simulink model "PTControl"  (Simulink 10.3)
settings: Solver=ode45  StartTime=0.0  StopTime=inf  RelTol=1e-3  EnableMultiTasking=on
(part 2 of 5)

== system PTControl/CarMaker/IPG Vehicle/CarAndTrailer/Forces/Tires ==
  note: The TireXX_Out signals will only be used if FileIdent is "CarMaker-Tire-CM4SL" in the tire parameter file!
      | An example parameter file can be found in Data/Tire/DT_CM4SL_UserTire.
  Sync_In : Inport
  TireFL_In : Inport  Port=2
  TireFR_In : Inport  Port=3
  TireRL_In : Inport  Port=4
  TireRR_In : Inport  Port=5
  Bus Creator{1..4} (4 alike) : BusCreator  Inputs=11
  Demux{1..3,8} (4 alike) : Demux  Outputs=7
      settings: DisplayOption=none
  TireFL : Subsystem
  TireFR : Subsystem
  TireRL : Subsystem
  TireRR : Subsystem
  TireFL_Out : Outport  VectorParamsAs1DForOutWhenUnconnected=off
  TireFR_Out : Outport  Port=2  VectorParamsAs1DForOutWhenUnconnected=off
  TireRL_Out : Outport  Port=3  VectorParamsAs1DForOutWhenUnconnected=off
  TireRR_Out : Outport  Port=4  VectorParamsAs1DForOutWhenUnconnected=off
  wires:
  Sync_In/1 -> TireRR/1(Sync_In), TireRL/1(Sync_In), TireFR/1(Sync_In), TireFL/1(Sync_In)
  Bus Creator4/1 -> TireRR_Out/1
  Bus Creator2/1 -> TireRL_Out/1
  Bus Creator1/1 -> TireFR_Out/1
  Demux3/5 -> TireRR/6(Rim_turnv)  "Tire_In Rim_turnv"
  Demux3/4 -> TireRR/5(Rim_rotv)  "Tire_In Rim_rotv"
  Demux3/1 -> TireRR/2(Load)  "Tire_In Load"
  Demux3/7 -> TireRR/8(muRoad)  "Tire_In mu"
  Demux3/6 -> TireRR/7(InclinAngle)  "Tire_In Camber"
  Demux3/2 -> TireRR/3(vxtrans)  "Tire_In vxtrans"
  Demux3/3 -> TireRR/4(vytrans)  "Tire_In vytrans"
  TireRR/11(AlignTrq) -> Bus Creator4/11  "Tire_Out AlignTrq"
  TireRR/10(RollResist) -> Bus Creator4/10  "Tire_Out RollResist"
  TireRR/9(OverturnTrq) -> Bus Creator4/9  "Tire_Out OverturnTrq"
  TireRR/8(LoadFrc) -> Bus Creator4/8  "Tire_Out LoadFrc"
  TireRR/7(SideFrc) -> Bus Creator4/7  "Tire_Out SideFrc"
  TireRR/6(LongFrc) -> Bus Creator4/6  "Tire_Out LongFrc"
  TireRR/5(vBelt) -> Bus Creator4/5  "Tire_Out vBelt"
  TireRR/4(rBelt_eff) -> Bus Creator4/4  "Tire_Out rBelt_eff"
  TireRR/3(TurnSlp) -> Bus Creator4/3  "Tire_Out TurnSlp"
  TireRR/1(Slp) -> Bus Creator4/1  "Tire_Out Slp"
  TireRR/2(Alpha) -> Bus Creator4/2  "Tire_Out Alpha"
  Demux2/5 -> TireRL/6(Rim_turnv)  "Tire_In Rim_turnv"
  Demux2/4 -> TireRL/5(Rim_rotv)  "Tire_In Rim_rotv"
  Demux2/1 -> TireRL/2(Load)  "Tire_In Load"
  Demux2/7 -> TireRL/8(muRoad)  "Tire_In mu"
  Demux2/6 -> TireRL/7(InclinAngle)  "Tire_In Camber"
  Demux2/2 -> TireRL/3(vxtrans)  "Tire_In vxtrans"
  Demux2/3 -> TireRL/4(vytrans)  "Tire_In vytrans"
  TireRL/11(AlignTrq) -> Bus Creator2/11  "Tire_Out AlignTrq"
  TireRL/10(RollResist) -> Bus Creator2/10  "Tire_Out RollResist"
  TireRL/9(OverturnTrq) -> Bus Creator2/9  "Tire_Out OverturnTrq"
  TireRL/8(LoadFrc) -> Bus Creator2/8  "Tire_Out LoadFrc"
  TireRL/7(SideFrc) -> Bus Creator2/7  "Tire_Out SideFrc"
  TireRL/6(LongFrc) -> Bus Creator2/6  "Tire_Out LongFrc"
  TireRL/5(vBelt) -> Bus Creator2/5  "Tire_Out vBelt"
  TireRL/4(rBelt_eff) -> Bus Creator2/4  "Tire_Out rBelt_eff"
  TireRL/3(TurnSlp) -> Bus Creator2/3  "Tire_Out TurnSlp"
  TireRL/1(Slp) -> Bus Creator2/1  "Tire_Out Slp"
  TireRL/2(Alpha) -> Bus Creator2/2  "Tire_Out Alpha"
  Demux1/5 -> TireFR/6(Rim_turnv)  "Tire_In Rim_turnv"
  Demux1/4 -> TireFR/5(Rim_rotv)  "Tire_In Rim_rotv"
  Demux1/1 -> TireFR/2(Load)  "Tire_In Load"
  Demux1/7 -> TireFR/8(muRoad)  "Tire_In mu"
  Demux1/6 -> TireFR/7(InclinAngle)  "Tire_In Camber"
  Demux1/2 -> TireFR/3(vxtrans)  "Tire_In vxtrans"
  Demux1/3 -> TireFR/4(vytrans)  "Tire_In vytrans"
  TireFR/11(AlignTrq) -> Bus Creator1/11  "Tire_Out AlignTrq"
  TireFR/10(RollResist) -> Bus Creator1/10  "Tire_Out RollResist"
  TireFR/9(OverturnTrq) -> Bus Creator1/9  "Tire_Out OverturnTrq"
  TireFR/8(LoadFrc) -> Bus Creator1/8  "Tire_Out LoadFrc"
  TireFR/7(SideFrc) -> Bus Creator1/7  "Tire_Out SideFrc"
  TireFR/6(LongFrc) -> Bus Creator1/6  "Tire_Out LongFrc"
  TireFR/5(vBelt) -> Bus Creator1/5  "Tire_Out vBelt"
  TireFR/4(rBelt_eff) -> Bus Creator1/4  "Tire_Out rBelt_eff"
  TireFR/3(TurnSlp) -> Bus Creator1/3  "Tire_Out TurnSlp"
  TireFR/1(Slp) -> Bus Creator1/1  "Tire_Out Slp"
  TireFR/2(Alpha) -> Bus Creator1/2  "Tire_Out Alpha"
  Demux8/5 -> TireFL/6(Rim_turnv)  "Tire_In Rim_turnv"
  Demux8/4 -> TireFL/5(Rim_rotv)  "Tire_In Rim_rotv"
  TireFL_In/1 -> Demux8/1
  Demux8/1 -> TireFL/2(Load)  "Tire_In Load"
  Demux8/7 -> TireFL/8(muRoad)  "Tire_In mu"
  Demux8/6 -> TireFL/7(InclinAngle)  "Tire_In Camber"
  Demux8/2 -> TireFL/3(vxtrans)  "Tire_In vxtrans"
  Demux8/3 -> TireFL/4(vytrans)  "Tire_In vytrans"
  TireFL/11(AlignTrq) -> Bus Creator3/11  "Tire_Out AlignTrq"
  TireFL/10(RollResist) -> Bus Creator3/10  "Tire_Out RollResist"
  TireFL/9(OverturnTrq) -> Bus Creator3/9  "Tire_Out OverturnTrq"
  TireFL/8(LoadFrc) -> Bus Creator3/8  "Tire_Out LoadFrc"
  TireFL/7(SideFrc) -> Bus Creator3/7  "Tire_Out SideFrc"
  TireFL/6(LongFrc) -> Bus Creator3/6  "Tire_Out LongFrc"
  TireFL/5(vBelt) -> Bus Creator3/5  "Tire_Out vBelt"
  TireFL/4(rBelt_eff) -> Bus Creator3/4  "Tire_Out rBelt_eff"
  TireFL/3(TurnSlp) -> Bus Creator3/3  "Tire_Out TurnSlp"
  TireFL/1(Slp) -> Bus Creator3/1  "Tire_Out Slp"
  TireFL/2(Alpha) -> Bus Creator3/2  "Tire_Out Alpha"
  Bus Creator3/1 -> TireFL_Out/1
  TireFR_In/1 -> Demux1/1
  TireRL_In/1 -> Demux2/1
  TireRR_In/1 -> Demux3/1

== system PTControl/CarMaker/IPG Vehicle/CarAndTrailer/Forces/Vehicle Forces ==
  Sync_In : Inport
  Bus Creator1 : BusCreator  Inputs=12
  Bus Creator8 : BusCreator  Inputs=16
  BusCreator1 : BusCreator  Inputs=4
  BusCreator2 : BusCreator  Inputs=9
  Demux : Demux  Outputs=16
      settings: DisplayOption=none
  Demux1 : Demux  Outputs=12
      settings: DisplayOption=none
  Demux2 : Demux  Outputs=13
      settings: DisplayOption=none
  Forces : S-Function  FunctionName=CM_Sfun  Parameters='Forces'  SFunctionDeploymentMode=off  EnableBusSupport=off
  Terminator : Terminator
  Sync_Out : Outport  VectorParamsAs1DForOutWhenUnconnected=off
  Car.Virtual : Outport  Port=2  VectorParamsAs1DForOutWhenUnconnected=off
  Car.Aero : Outport  Port=3  VectorParamsAs1DForOutWhenUnconnected=off
  Car.Load : Outport  Port=4  VectorParamsAs1DForOutWhenUnconnected=off
  wires:
  BusCreator1/1 -> Terminator/1  "Aero IF (in)"
  Demux2/13 -> BusCreator2/9  "car Aero Trq_1 z"
  Demux2/12 -> BusCreator2/8  "car Aero Trq_1 y"
  Demux2/11 -> BusCreator2/7  "car Aero Trq_1 x"
  Demux2/10 -> BusCreator2/6  "car Aero Frc_1 z"
  Demux2/9 -> BusCreator2/5  "car Aero Frc_1 y"
  Demux2/8 -> BusCreator2/4  "car Aero Frc_1 x"
  Demux2/7 -> BusCreator2/3  "car Aero PoA_1 z"
  Demux2/6 -> BusCreator2/2  "car Aero PoA_1 y"
  Demux2/5 -> BusCreator2/1  "car Aero PoA_1 x"
  Demux2/4 -> BusCreator1/4  "car Aero tau_1"
  Demux2/3 -> BusCreator1/3  "car Aero ApproachVel_1 z"
  Demux2/2 -> BusCreator1/2  "car Aero ApproachVel_1 y"
  Demux2/1 -> BusCreator1/1  "car Aero ApproachVel_1 x"
  Demux/16 -> Bus Creator8/16  "Car Load_3 tz"
  Demux/15 -> Bus Creator8/15  "Car Load_3 ty"
  Demux/14 -> Bus Creator8/14  "Car Load_3 tx"
  Demux/13 -> Bus Creator8/13  "Car Load_3 mass"
  Demux1/12 -> Bus Creator1/12  "Car Virtual Trq_0 z"
  Demux1/11 -> Bus Creator1/11  "Car Virtual Trq_0 y"
  Demux1/10 -> Bus Creator1/10  "Car Virtual Trq_0 x"
  Demux1/9 -> Bus Creator1/9  "Car Virtual Trq_1 z"
  Demux1/8 -> Bus Creator1/8  "Car Virtual Trq_1 y"
  Demux1/7 -> Bus Creator1/7  "Car Virtual Trq_1 x"
  Demux1/6 -> Bus Creator1/6  "Car Virtual Frc_0 z"
  Demux1/5 -> Bus Creator1/5  "Car Virtual Frc_0 y"
  Demux1/4 -> Bus Creator1/4  "Car Virtual Frc_0 x"
  Sync_In/1 -> Forces/1
  Forces/1 -> Sync_Out/1
  BusCreator2/1 -> Car.Aero/1
  Demux1/1 -> Bus Creator1/1  "Car Virtual Frc_1 x"
  Demux1/2 -> Bus Creator1/2  "Car Virtual Frc_1 y"
  Demux1/3 -> Bus Creator1/3  "Car Virtual Frc_1 z"
  Forces/3 -> Demux2/1
  Forces/2 -> Demux1/1
  Bus Creator1/1 -> Car.Virtual/1
  Bus Creator8/1 -> Car.Load/1
  Demux/1 -> Bus Creator8/1  "Car Load_0 mass"
  Demux/2 -> Bus Creator8/2  "Car Load_0 tx"
  Demux/3 -> Bus Creator8/3  "Car Load_0 ty"
  Demux/4 -> Bus Creator8/4  "Car Load_0 tz"
  Demux/5 -> Bus Creator8/5  "Car Load_1 mass"
  Demux/6 -> Bus Creator8/6  "Car Load_1 tx"
  Demux/7 -> Bus Creator8/7  "Car Load_1 ty"
  Demux/8 -> Bus Creator8/8  "Car Load_1 tz"
  Demux/9 -> Bus Creator8/9  "Car Load_2 mass"
  Demux/10 -> Bus Creator8/10  "Car Load_2 tx"
  Demux/11 -> Bus Creator8/11  "Car Load_2 ty"
  Demux/12 -> Bus Creator8/12  "Car Load_2 tz"
  Forces/4 -> Demux/1

== system PTControl/CarMaker/IPG Vehicle/CarAndTrailer/Trailer/CreateBus Car.Hitch.FrcTrq ==
  In1 : Inport
  Bus Creator7 : BusCreator  Inputs=6
  Demux7 : Demux  Outputs=6
      settings: DisplayOption=none
  Out1 : Outport  VectorParamsAs1DForOutWhenUnconnected=off
  wires:
  In1/1 -> Demux7/1
  Bus Creator7/1 -> Out1/1
  Demux7/6 -> Bus Creator7/6  "Car Hitch Trq2Car z"
  Demux7/5 -> Bus Creator7/5  "Car Hitch Trq2Car y"
  Demux7/4 -> Bus Creator7/4  "Car Hitch Trq2Car x"
  Demux7/3 -> Bus Creator7/3  "Car Hitch Frc2Car z"
  Demux7/2 -> Bus Creator7/2  "Car Hitch Frc2Car y"
  Demux7/1 -> Bus Creator7/1  "Car Hitch Frc2Car x"

== system PTControl/CarMaker/IPG Vehicle/CarAndTrailer/Trailer/CreateBus Vhcl.Motion ==
  In1 : Inport
  BusCreator : BusCreator  Inputs=15
  Demux : Demux  Outputs=15
      settings: DisplayOption=none
  Out1 : Outport  VectorParamsAs1DForOutWhenUnconnected=off
  wires:
  Demux/15 -> BusCreator/15  "Vhcl YawAcc"
  Demux/14 -> BusCreator/14  "Vhcl YawVel"
  Demux/13 -> BusCreator/13  "Vhcl Yaw"
  Demux/12 -> BusCreator/12  "Vhcl PitchAcc"
  Demux/11 -> BusCreator/11  "Vhcl PitchVel"
  Demux/10 -> BusCreator/10  "Vhcl Pitch"
  Demux/9 -> BusCreator/9  "Vhcl RollAcc"
  Demux/8 -> BusCreator/8  "Vhcl RollVel"
  Demux/7 -> BusCreator/7  "Vhcl Roll"
  Demux/6 -> BusCreator/6  "Vhcl Hitch_Pos z"
  Demux/5 -> BusCreator/5  "Vhcl Hitch_Pos y"
  Demux/4 -> BusCreator/4  "Vhcl Hitch_Pos x"
  Demux/3 -> BusCreator/3  "Vhcl sRoad"
  Demux/2 -> BusCreator/2  "Vhcl Distance"
  Demux/1 -> BusCreator/1  "Vhcl v"
  In1/1 -> Demux/1
  BusCreator/1 -> Out1/1

== system PTControl/CarMaker/IPG Vehicle/CarAndTrailer/Trailer/CreateBus Vhcl.PoI ==
  In1 : Inport
  Bus Creator3 : BusCreator  Inputs=18
  Demux3 : Demux  Outputs=18
      settings: DisplayOption=none
  Out1 : Outport  VectorParamsAs1DForOutWhenUnconnected=off
  wires:
  Demux3/18 -> Bus Creator3/18  "Vhcl PoI_GCS Elev"
  Demux3/17 -> Bus Creator3/17  "Vhcl PoI_GCS Lat"
  Demux3/16 -> Bus Creator3/16  "Vhcl PoI_GCS Long"
  Demux3/15 -> Bus Creator3/15  "Vhcl PoI_Acc_1 z"
  Demux3/14 -> Bus Creator3/14  "Vhcl PoI_Acc_1 y"
  Demux3/13 -> Bus Creator3/13  "Vhcl PoI_Acc_1 x"
  Demux3/12 -> Bus Creator3/12  "Vhcl PoI_Vel_1 z"
  Demux3/11 -> Bus Creator3/11  "Vhcl PoI_Vel_1 y"
  Demux3/10 -> Bus Creator3/10  "Vhcl PoI_Vel_1 x"
  Demux3/9 -> Bus Creator3/9  "Vhcl PoI_Acc z"
  Demux3/8 -> Bus Creator3/8  "Vhcl PoI_Acc y"
  Demux3/7 -> Bus Creator3/7  "Vhcl PoI_Acc x"
  Demux3/6 -> Bus Creator3/6  "Vhcl PoI_Vel z"
  Demux3/5 -> Bus Creator3/5  "Vhcl PoI_Vel y"
  Demux3/4 -> Bus Creator3/4  "Vhcl PoI_Vel x"
  Demux3/3 -> Bus Creator3/3  "Vhcl PoI_Pos z"
  Demux3/2 -> Bus Creator3/2  "Vhcl PoI_Pos y"
  In1/1 -> Demux3/1
  Bus Creator3/1 -> Out1/1
  Demux3/1 -> Bus Creator3/1  "Vhcl PoI_Pos x"

== system PTControl/CarMaker/IPG Vehicle/CarAndTrailer/Trailer/CreateBus Vhcl.Steering ==
  In1 : Inport
  Bus Creator3 : BusCreator  Inputs=4
  Demux : Demux
      settings: DisplayOption=none
  Out1 : Outport  VectorParamsAs1DForOutWhenUnconnected=off
  wires:
  Bus Creator3/1 -> Out1/1
  Demux/1 -> Bus Creator3/1  "Vhcl Steering Ang"
  Demux/3 -> Bus Creator3/3  "Vhcl Steering AngAcc"
  Demux/2 -> Bus Creator3/2  "Vhcl Steering AngVel"
  Demux/4 -> Bus Creator3/4  "Vhcl Steering Trq"
  In1/1 -> Demux/1

== system PTControl/CarMaker/IPG Vehicle/CarAndTrailer/Trailer/CreateBus Vhcl.Wheel.FL ==
  In1 : Inport
  Bus Creator3 : BusCreator  Inputs=14
  Demux3 : Demux  Outputs=14
      settings: DisplayOption=none
  Out1 : Outport  VectorParamsAs1DForOutWhenUnconnected=off
  wires:
  Demux3/14 -> Bus Creator3/14  "Vhcl Wheel FL Trq_WhlBearing"
  Demux3/13 -> Bus Creator3/13  "Vhcl Wheel FL Trq_T2W"
  Demux3/12 -> Bus Creator3/12  "Vhcl Wheel FL SideSlip"
  Demux3/11 -> Bus Creator3/11  "Vhcl Wheel FL LongSlip"
  Demux3/10 -> Bus Creator3/10  "Vhcl Wheel FL vBelt"
  Demux3/9 -> Bus Creator3/9  "Vhcl Wheel FL Fz"
  Demux3/8 -> Bus Creator3/8  "Vhcl Wheel FL Fy"
  Demux3/7 -> Bus Creator3/7  "Vhcl Wheel FL Fx"
  Demux3/6 -> Bus Creator3/6  "Vhcl Wheel FL r_zxy z"
  Demux3/5 -> Bus Creator3/5  "Vhcl Wheel FL r_zxy y"
  Demux3/4 -> Bus Creator3/4  "Vhcl Wheel FL r_zxy x"
  Demux3/3 -> Bus Creator3/3  "Vhcl Wheel FL t z"
  Demux3/2 -> Bus Creator3/2  "Vhcl Wheel FL t y"
  In1/1 -> Demux3/1
  Bus Creator3/1 -> Out1/1
  Demux3/1 -> Bus Creator3/1  "Vhcl Wheel FL t x"

== system PTControl/CarMaker/IPG Vehicle/CarAndTrailer/Trailer/CreateBus Vhcl.Wheel.FR ==
  In1 : Inport
  Bus Creator3 : BusCreator  Inputs=14
  Demux3 : Demux  Outputs=14
      settings: DisplayOption=none
  Out1 : Outport  VectorParamsAs1DForOutWhenUnconnected=off
  wires:
  Demux3/14 -> Bus Creator3/14  "Vhcl Wheel FR Trq_WhlBearing"
  Demux3/13 -> Bus Creator3/13  "Vhcl Wheel FR Trq_T2W"
  Demux3/12 -> Bus Creator3/12  "Vhcl Wheel FR SideSlip"
  Demux3/11 -> Bus Creator3/11  "Vhcl Wheel FR LongSlip"
  Demux3/10 -> Bus Creator3/10  "Vhcl Wheel FR vBelt"
  Demux3/9 -> Bus Creator3/9  "Vhcl Wheel FR Fz"
  Demux3/8 -> Bus Creator3/8  "Vhcl Wheel FR Fy"
  Demux3/7 -> Bus Creator3/7  "Vhcl Wheel FR Fx"
  Demux3/6 -> Bus Creator3/6  "Vhcl Wheel FR r_zxy z"
  Demux3/5 -> Bus Creator3/5  "Vhcl Wheel FR r_zxy y"
  Demux3/4 -> Bus Creator3/4  "Vhcl Wheel FR r_zxy x"
  Demux3/3 -> Bus Creator3/3  "Vhcl Wheel FR t z"
  Demux3/2 -> Bus Creator3/2  "Vhcl Wheel FR t y"
  In1/1 -> Demux3/1
  Bus Creator3/1 -> Out1/1
  Demux3/1 -> Bus Creator3/1  "Vhcl Wheel FR t x"

== system PTControl/CarMaker/IPG Vehicle/CarAndTrailer/Trailer/CreateBus Vhcl.Wheel.RL ==
  In1 : Inport
  Bus Creator3 : BusCreator  Inputs=14
  Demux3 : Demux  Outputs=14
      settings: DisplayOption=none
  Out1 : Outport  VectorParamsAs1DForOutWhenUnconnected=off
  wires:
  Demux3/14 -> Bus Creator3/14  "Vhcl Wheel RL Trq_WhlBearing"
  Demux3/13 -> Bus Creator3/13  "Vhcl Wheel RL Trq_T2W"
  Demux3/12 -> Bus Creator3/12  "Vhcl Wheel RL SideSlip"
  Demux3/11 -> Bus Creator3/11  "Vhcl Wheel RL LongSlip"
  Demux3/10 -> Bus Creator3/10  "Vhcl Wheel RL vBelt"
  Demux3/9 -> Bus Creator3/9  "Vhcl Wheel RL Fz"
  Demux3/8 -> Bus Creator3/8  "Vhcl Wheel RL Fy"
  Demux3/7 -> Bus Creator3/7  "Vhcl Wheel RL Fx"
  Demux3/6 -> Bus Creator3/6  "Vhcl Wheel RL r_zxy z"
  Demux3/5 -> Bus Creator3/5  "Vhcl Wheel RL r_zxy y"
  Demux3/4 -> Bus Creator3/4  "Vhcl Wheel RL r_zxy x"
  Demux3/3 -> Bus Creator3/3  "Vhcl Wheel RL t z"
  Demux3/2 -> Bus Creator3/2  "Vhcl Wheel RL t y"
  In1/1 -> Demux3/1
  Bus Creator3/1 -> Out1/1
  Demux3/1 -> Bus Creator3/1  "Vhcl Wheel RL t x"

== system PTControl/CarMaker/IPG Vehicle/CarAndTrailer/Trailer/CreateBus Vhcl.Wheel.RR ==
  In1 : Inport
  Bus Creator3 : BusCreator  Inputs=14
  Demux3 : Demux  Outputs=14
      settings: DisplayOption=none
  Out1 : Outport  VectorParamsAs1DForOutWhenUnconnected=off
  wires:
  Demux3/14 -> Bus Creator3/14  "Vhcl Wheel RR Trq_WhlBearing"
  Demux3/13 -> Bus Creator3/13  "Vhcl Wheel RR Trq_T2W"
  Demux3/12 -> Bus Creator3/12  "Vhcl Wheel RR SideSlip"
  Demux3/11 -> Bus Creator3/11  "Vhcl Wheel RR LongSlip"
  Demux3/10 -> Bus Creator3/10  "Vhcl Wheel RR vBelt"
  Demux3/9 -> Bus Creator3/9  "Vhcl Wheel RR Fz"
  Demux3/8 -> Bus Creator3/8  "Vhcl Wheel RR Fy"
  Demux3/7 -> Bus Creator3/7  "Vhcl Wheel RR Fx"
  Demux3/6 -> Bus Creator3/6  "Vhcl Wheel RR r_zxy z"
  Demux3/5 -> Bus Creator3/5  "Vhcl Wheel RR r_zxy y"
  Demux3/4 -> Bus Creator3/4  "Vhcl Wheel RR r_zxy x"
  Demux3/3 -> Bus Creator3/3  "Vhcl Wheel RR t z"
  Demux3/2 -> Bus Creator3/2  "Vhcl Wheel RR t y"
  In1/1 -> Demux3/1
  Bus Creator3/1 -> Out1/1
  Demux3/1 -> Bus Creator3/1  "Vhcl Wheel RR t x"

== system PTControl/CarMaker/IPG Vehicle/PowerTrain/PTControl Example/CreateBus PTC BatteryHVOut ==
  In : Inport
  BusCreator : BusCreator  Inputs=2
  Demux : Demux  Outputs=2
      settings: DisplayOption=none
  Out : Outport  VectorParamsAs1DForOutWhenUnconnected=off
  wires:
  Demux/2 -> BusCreator/2  "PTC BattHVOut MassFlowCool_trg"
  Demux/1 -> BusCreator/1  "PTC BattHVOut Temp_trg"
  In/1 -> Demux/1
  BusCreator/1 -> Out/1

== system PTControl/CarMaker/IPG Vehicle/PowerTrain/PTControl Example/CreateBus PTC BatteryLVOut ==
  In : Inport
  BusCreator : BusCreator  Inputs=2
  Demux : Demux  Outputs=2
      settings: DisplayOption=none
  Out : Outport  VectorParamsAs1DForOutWhenUnconnected=off
  wires:
  Demux/2 -> BusCreator/2  "PTC BattLVOut MassFlowCool_trg"
  In/1 -> Demux/1
  Demux/1 -> BusCreator/1  "PTC BattLVOut Temp_trg"
  BusCreator/1 -> Out/1

== system PTControl/CarMaker/IPG Vehicle/PowerTrain/PTControl Example/CreateBus PTC EngineOut ==
  In : Inport
  BusCreator : BusCreator  Inputs=5
  Demux : Demux  Outputs=5
      settings: DisplayOption=none
  Out : Outport  VectorParamsAs1DForOutWhenUnconnected=off
  wires:
  Demux/5 -> BusCreator/5  "PTC EngineOut rotv_trg"
  Demux/4 -> BusCreator/4  "PTC EngineOut Trq_trg"
  Demux/3 -> BusCreator/3  "PTC EngineOut Load"
  Demux/2 -> BusCreator/2  "PTC EngineOut FuelCutOff"
  Demux/1 -> BusCreator/1  "PTC EngineOut set_ISC"
  BusCreator/1 -> Out/1
  In/1 -> Demux/1

== system PTControl/CarMaker/IPG Vehicle/PowerTrain/PTControl Example/CreateBus PTC ISGOut ==
  In : Inport
  BusCreator : BusCreator  Inputs=3
  Demux : Demux  Outputs=3
      settings: DisplayOption=none
  Out : Outport  VectorParamsAs1DForOutWhenUnconnected=off
  wires:
  Demux/3 -> BusCreator/3  "PTC ISGOut rotv_trg"
  Demux/2 -> BusCreator/2  "PTC ISGOut Trq_trg"
  Demux/1 -> BusCreator/1  "PTC ISGOut Load"
  BusCreator/1 -> Out/1
  In/1 -> Demux/1

== system PTControl/CarMaker/IPG Vehicle/PowerTrain/PTControl Example/CreateBus PTC MiscOut ==
  In : Inport
  BusCreator : BusCreator  Inputs=4
  Demux : Demux
      settings: DisplayOption=none
  Out : Outport  VectorParamsAs1DForOutWhenUnconnected=off
  wires:
  Demux/4 -> BusCreator/4  "PTC_Out Ignition"
  Demux/3 -> BusCreator/3  "PTC_Out StrategyMode"
  Demux/2 -> BusCreator/2  "PTC_Out OperationError"
  Demux/1 -> BusCreator/1  "PTC_Out OperationState"
  BusCreator/1 -> Out/1
  In/1 -> Demux/1

== system PTControl/CarMaker/IPG Vehicle/PowerTrain/PTControl Example/CreateBus PTC PwrSupplyOut ==
  In : Inport
  BusCreator : BusCreator  Inputs=1
  Demux : Demux  Outputs=1
      settings: DisplayOption=none
  Out : Outport  VectorParamsAs1DForOutWhenUnconnected=off
  wires:
  Demux/1 -> BusCreator/1  "PTC PwrSupplyOut Pwr_HV1toLV_trg"
  BusCreator/1 -> Out/1
  In/1 -> Demux/1

== system PTControl/CarMaker/IPG Vehicle/PowerTrain/PTControl Example/CreateBus PTC WheelOut ==
  In : Inport
  BusCreator : BusCreator  Inputs=8
  Demux : Demux  Outputs=8
      settings: DisplayOption=none
  Out : Outport  VectorParamsAs1DForOutWhenUnconnected=off
  wires:
  Demux/8 -> BusCreator/8  "PTC WheelOut_RR Trq_BrakeReg_max"
  Demux/7 -> BusCreator/7  "PTC WheelOut_RR Trq_BrakeReg"
  Demux/6 -> BusCreator/6  "PTC WheelOut_RL Trq_BrakeReg_max"
  Demux/5 -> BusCreator/5  "PTC WheelOut_RL Trq_BrakeReg"
  Demux/4 -> BusCreator/4  "PTC WheelOut_FR Trq_BrakeReg_max"
  Demux/3 -> BusCreator/3  "PTC WheelOut_FR Trq_BrakeReg"
  Demux/2 -> BusCreator/2  "PTC WheelOut_FL Trq_BrakeReg_max"
  Demux/1 -> BusCreator/1  "PTC WheelOut_FL Trq_BrakeReg"
  BusCreator/1 -> Out/1
  In/1 -> Demux/1

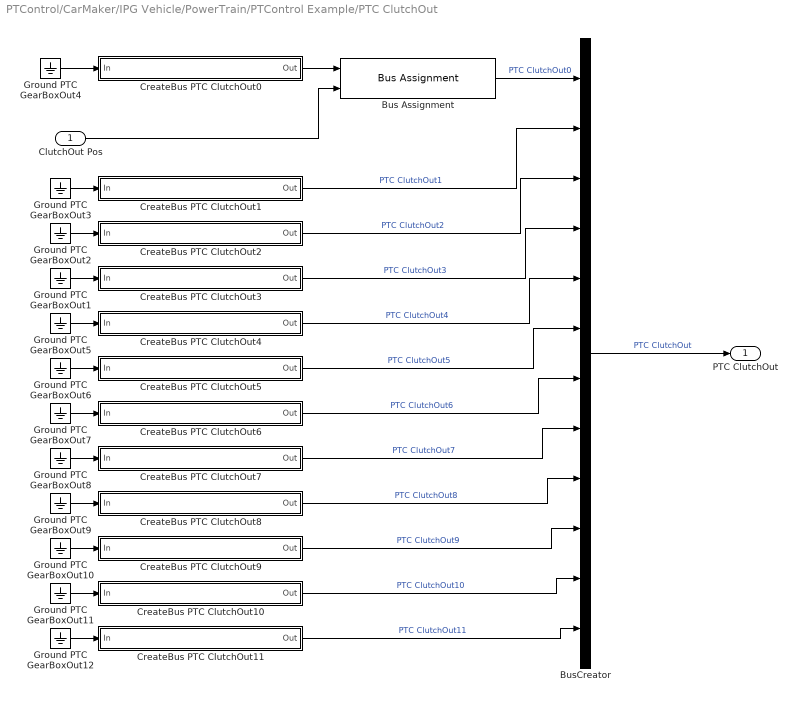
== system PTControl/CarMaker/IPG Vehicle/PowerTrain/PTControl Example/PTC ClutchOut ==
  ClutchOut Pos : Inport
  Bus Assignment : BusAssignment  AssignedSignals=PTC ClutchOut0 Pos
  BusCreator : BusCreator  Inputs=12
  CreateBus PTC ClutchOut0 : Subsystem
  CreateBus PTC ClutchOut1 : Subsystem
  CreateBus PTC ClutchOut10 : Subsystem
  CreateBus PTC ClutchOut11 : Subsystem
  CreateBus PTC ClutchOut2 : Subsystem
  CreateBus PTC ClutchOut3 : Subsystem
  CreateBus PTC ClutchOut4 : Subsystem
  CreateBus PTC ClutchOut5 : Subsystem
  CreateBus PTC ClutchOut6 : Subsystem
  CreateBus PTC ClutchOut7 : Subsystem
  CreateBus PTC ClutchOut8 : Subsystem
  CreateBus PTC ClutchOut9 : Subsystem
  Ground PTC GearBoxOut{1..12} (12 alike) : Ground
  PTC ClutchOut : Outport
  wires:
  ClutchOut Pos/1 -> Bus Assignment/2
  CreateBus PTC ClutchOut0/1(Out) -> Bus Assignment/1
  Ground PTC GearBoxOut4/1 -> CreateBus PTC ClutchOut0/1(In)
  Ground PTC GearBoxOut3/1 -> CreateBus PTC ClutchOut1/1(In)
  Ground PTC GearBoxOut2/1 -> CreateBus PTC ClutchOut2/1(In)
  Ground PTC GearBoxOut1/1 -> CreateBus PTC ClutchOut3/1(In)
  Ground PTC GearBoxOut5/1 -> CreateBus PTC ClutchOut4/1(In)
  Ground PTC GearBoxOut6/1 -> CreateBus PTC ClutchOut5/1(In)
  Ground PTC GearBoxOut7/1 -> CreateBus PTC ClutchOut6/1(In)
  Ground PTC GearBoxOut8/1 -> CreateBus PTC ClutchOut7/1(In)
  Ground PTC GearBoxOut9/1 -> CreateBus PTC ClutchOut8/1(In)
  Ground PTC GearBoxOut10/1 -> CreateBus PTC ClutchOut9/1(In)
  Ground PTC GearBoxOut11/1 -> CreateBus PTC ClutchOut10/1(In)
  Ground PTC GearBoxOut12/1 -> CreateBus PTC ClutchOut11/1(In)
  Bus Assignment/1 -> BusCreator/1  "PTC ClutchOut0"
  CreateBus PTC ClutchOut1/1(Out) -> BusCreator/2  "PTC ClutchOut1"
  CreateBus PTC ClutchOut2/1(Out) -> BusCreator/3  "PTC ClutchOut2"
  CreateBus PTC ClutchOut3/1(Out) -> BusCreator/4  "PTC ClutchOut3"
  CreateBus PTC ClutchOut4/1(Out) -> BusCreator/5  "PTC ClutchOut4"
  CreateBus PTC ClutchOut5/1(Out) -> BusCreator/6  "PTC ClutchOut5"
  CreateBus PTC ClutchOut6/1(Out) -> BusCreator/7  "PTC ClutchOut6"
  CreateBus PTC ClutchOut7/1(Out) -> BusCreator/8  "PTC ClutchOut7"
  CreateBus PTC ClutchOut8/1(Out) -> BusCreator/9  "PTC ClutchOut8"
  CreateBus PTC ClutchOut9/1(Out) -> BusCreator/10  "PTC ClutchOut9"
  CreateBus PTC ClutchOut10/1(Out) -> BusCreator/11  "PTC ClutchOut10"
  CreateBus PTC ClutchOut11/1(Out) -> BusCreator/12  "PTC ClutchOut11"
  BusCreator/1 -> PTC ClutchOut/1  "PTC ClutchOut"

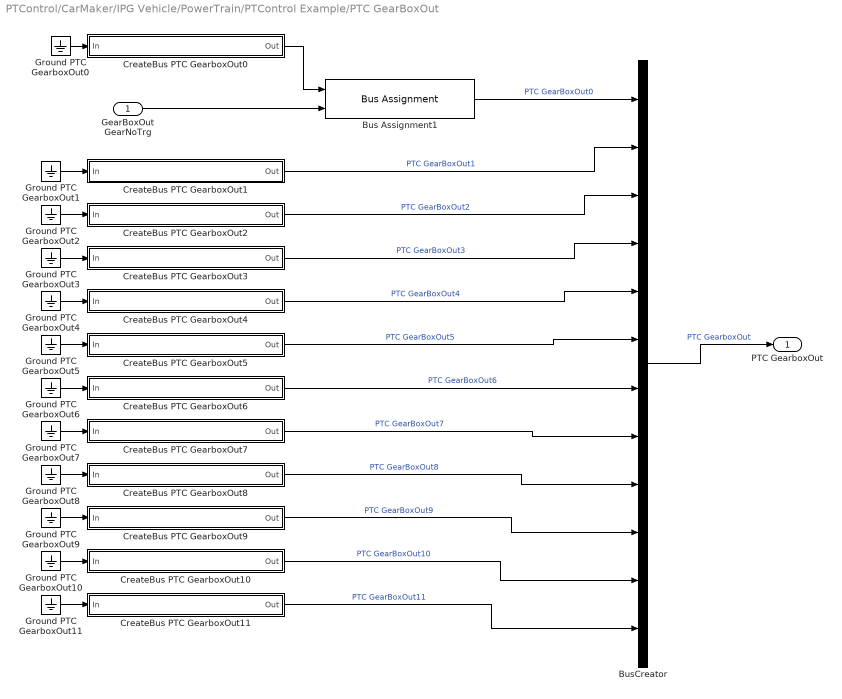
== system PTControl/CarMaker/IPG Vehicle/PowerTrain/PTControl Example/PTC GearBoxOut ==
  GearBoxOut GearNoTrg : Inport
  Bus Assignment1 : BusAssignment  AssignedSignals=PTC GearboxOut0 GearNoTrg
  BusCreator : BusCreator  Inputs=12
  CreateBus PTC GearboxOut0 : Subsystem
  CreateBus PTC GearboxOut1 : Subsystem
  CreateBus PTC GearboxOut10 : Subsystem
  CreateBus PTC GearboxOut11 : Subsystem
  CreateBus PTC GearboxOut2 : Subsystem
  CreateBus PTC GearboxOut3 : Subsystem
  CreateBus PTC GearboxOut4 : Subsystem
  CreateBus PTC GearboxOut5 : Subsystem
  CreateBus PTC GearboxOut6 : Subsystem
  CreateBus PTC GearboxOut7 : Subsystem
  CreateBus PTC GearboxOut8 : Subsystem
  CreateBus PTC GearboxOut9 : Subsystem
  Ground PTC GearboxOut{0..11} (12 alike) : Ground
  PTC GearboxOut : Outport
  wires:
  GearBoxOut GearNoTrg/1 -> Bus Assignment1/2
  Ground PTC GearboxOut0/1 -> CreateBus PTC GearboxOut0/1(In)
  CreateBus PTC GearboxOut0/1(Out) -> Bus Assignment1/1
  Ground PTC GearboxOut3/1 -> CreateBus PTC GearboxOut3/1(In)
  Ground PTC GearboxOut2/1 -> CreateBus PTC GearboxOut2/1(In)
  Ground PTC GearboxOut1/1 -> CreateBus PTC GearboxOut1/1(In)
  Ground PTC GearboxOut4/1 -> CreateBus PTC GearboxOut4/1(In)
  Ground PTC GearboxOut5/1 -> CreateBus PTC GearboxOut5/1(In)
  Ground PTC GearboxOut6/1 -> CreateBus PTC GearboxOut6/1(In)
  Ground PTC GearboxOut7/1 -> CreateBus PTC GearboxOut7/1(In)
  Ground PTC GearboxOut8/1 -> CreateBus PTC GearboxOut8/1(In)
  Ground PTC GearboxOut9/1 -> CreateBus PTC GearboxOut9/1(In)
  Ground PTC GearboxOut10/1 -> CreateBus PTC GearboxOut10/1(In)
  Ground PTC GearboxOut11/1 -> CreateBus PTC GearboxOut11/1(In)
  Bus Assignment1/1 -> BusCreator/1  "PTC GearBoxOut0"
  CreateBus PTC GearboxOut1/1(Out) -> BusCreator/2  "PTC GearBoxOut1"
  CreateBus PTC GearboxOut2/1(Out) -> BusCreator/3  "PTC GearBoxOut2"
  CreateBus PTC GearboxOut3/1(Out) -> BusCreator/4  "PTC GearBoxOut3"
  CreateBus PTC GearboxOut4/1(Out) -> BusCreator/5  "PTC GearBoxOut4"
  CreateBus PTC GearboxOut5/1(Out) -> BusCreator/6  "PTC GearBoxOut5"
  CreateBus PTC GearboxOut6/1(Out) -> BusCreator/7  "PTC GearBoxOut6"
  CreateBus PTC GearboxOut7/1(Out) -> BusCreator/8  "PTC GearBoxOut7"
  CreateBus PTC GearboxOut8/1(Out) -> BusCreator/9  "PTC GearBoxOut8"
  CreateBus PTC GearboxOut9/1(Out) -> BusCreator/10  "PTC GearBoxOut9"
  CreateBus PTC GearboxOut10/1(Out) -> BusCreator/11  "PTC GearBoxOut10"
  CreateBus PTC GearboxOut11/1(Out) -> BusCreator/12  "PTC GearBoxOut11"
  BusCreator/1 -> PTC GearboxOut/1  "PTC GearboxOut"

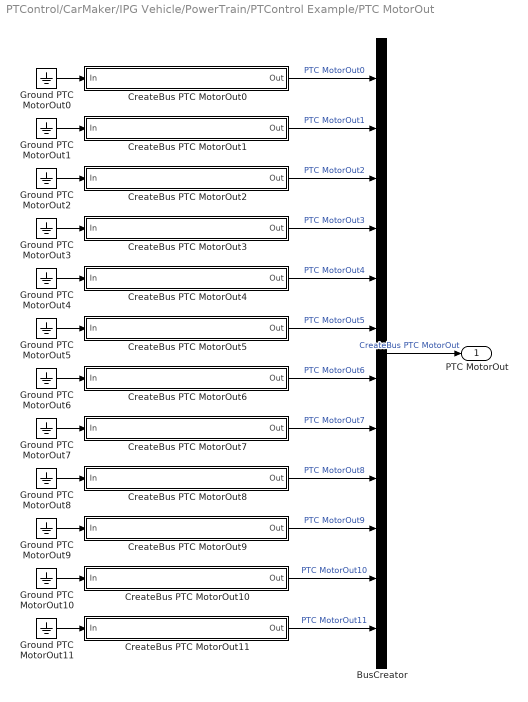
== system PTControl/CarMaker/IPG Vehicle/PowerTrain/PTControl Example/PTC MotorOut ==
  BusCreator : BusCreator  Inputs=12
  CreateBus PTC MotorOut0 : Subsystem
  CreateBus PTC MotorOut1 : Subsystem
  CreateBus PTC MotorOut10 : Subsystem
  CreateBus PTC MotorOut11 : Subsystem
  CreateBus PTC MotorOut2 : Subsystem
  CreateBus PTC MotorOut3 : Subsystem
  CreateBus PTC MotorOut4 : Subsystem
  CreateBus PTC MotorOut5 : Subsystem
  CreateBus PTC MotorOut6 : Subsystem
  CreateBus PTC MotorOut7 : Subsystem
  CreateBus PTC MotorOut8 : Subsystem
  CreateBus PTC MotorOut9 : Subsystem
  Ground PTC MotorOut{0..11} (12 alike) : Ground
  PTC MotorOut : Outport
  wires:
  CreateBus PTC MotorOut0/1(Out) -> BusCreator/1  "PTC MotorOut0"
  Ground PTC MotorOut0/1 -> CreateBus PTC MotorOut0/1(In)
  Ground PTC MotorOut3/1 -> CreateBus PTC MotorOut3/1(In)
  Ground PTC MotorOut1/1 -> CreateBus PTC MotorOut1/1(In)
  CreateBus PTC MotorOut1/1(Out) -> BusCreator/2  "PTC MotorOut1"
  Ground PTC MotorOut4/1 -> CreateBus PTC MotorOut4/1(In)
  Ground PTC MotorOut2/1 -> CreateBus PTC MotorOut2/1(In)
  CreateBus PTC MotorOut2/1(Out) -> BusCreator/3  "PTC MotorOut2"
  Ground PTC MotorOut5/1 -> CreateBus PTC MotorOut5/1(In)
  Ground PTC MotorOut6/1 -> CreateBus PTC MotorOut6/1(In)
  Ground PTC MotorOut7/1 -> CreateBus PTC MotorOut7/1(In)
  Ground PTC MotorOut8/1 -> CreateBus PTC MotorOut8/1(In)
  Ground PTC MotorOut9/1 -> CreateBus PTC MotorOut9/1(In)
  Ground PTC MotorOut10/1 -> CreateBus PTC MotorOut10/1(In)
  Ground PTC MotorOut11/1 -> CreateBus PTC MotorOut11/1(In)
  CreateBus PTC MotorOut4/1(Out) -> BusCreator/5  "PTC MotorOut4"
  CreateBus PTC MotorOut5/1(Out) -> BusCreator/6  "PTC MotorOut5"
  CreateBus PTC MotorOut6/1(Out) -> BusCreator/7  "PTC MotorOut6"
  CreateBus PTC MotorOut7/1(Out) -> BusCreator/8  "PTC MotorOut7"
  CreateBus PTC MotorOut8/1(Out) -> BusCreator/9  "PTC MotorOut8"
  CreateBus PTC MotorOut9/1(Out) -> BusCreator/10  "PTC MotorOut9"
  CreateBus PTC MotorOut10/1(Out) -> BusCreator/11  "PTC MotorOut10"
  CreateBus PTC MotorOut11/1(Out) -> BusCreator/12  "PTC MotorOut11"
  CreateBus PTC MotorOut3/1(Out) -> BusCreator/4  "PTC MotorOut3"
  BusCreator/1 -> PTC MotorOut/1  "CreateBus PTC MotorOut"

== system PTControl/CarMaker/IPG Vehicle/PowerTrain/PTControl Example/PTControl Example ==
  note: Minimalistic PTControl example model, that only works with
      | the 'Generic' powertrain and the 'Manual' gearbox.
  EngineIn : Inport
  VhclCtrl.PT : Inport  Port=2
  Bus Selector : BusSelector  OutputSignals=VhclCtrl Key,VhclCtrl Gas,VhclCtrl Clutch,VhclCtrl GearNo
  Bus Selector1 : BusSelector  OutputSignals=PTC EngineIn.PTC EngineIn Engine_on
  Engine : Subsystem
  ISG : Subsystem
  PTC : Subsystem
  PTC MiscOut : Outport  VectorParamsAs1DForOutWhenUnconnected=off
  EngineOut : Outport  Port=2  VectorParamsAs1DForOutWhenUnconnected=off
  ISGOut : Outport  Port=3  VectorParamsAs1DForOutWhenUnconnected=off
  ClutchOut Pos : Outport  Port=4  VectorParamsAs1DForOutWhenUnconnected=off
  GearBoxOut GearNoTrg : Outport  Port=5  VectorParamsAs1DForOutWhenUnconnected=off
  wires:
  VhclCtrl.PT/1 -> Bus Selector/1
  EngineIn/1 -> Bus Selector1/1
  Engine/1(EngineOut) -> EngineOut/1
  Bus Selector1/1 -> Engine/2(Engine_on), PTC/2(Engine_on)  "<PTC EngineIn Engine_on>"
  Bus Selector/2 -> Engine/1(Gas)  "<VhclCtrl Gas>"
  ISG/1(ISGOut) -> ISGOut/1
  PTC/1(PTC MiscOut) -> PTC MiscOut/1
  Bus Selector/4 -> GearBoxOut GearNoTrg/1  "<VhclCtrl GearNo>"
  Bus Selector/3 -> ClutchOut Pos/1  "<VhclCtrl Clutch>"
  Bus Selector/1 -> PTC/1(Key), ISG/1(Key)  "<VhclCtrl Key>"

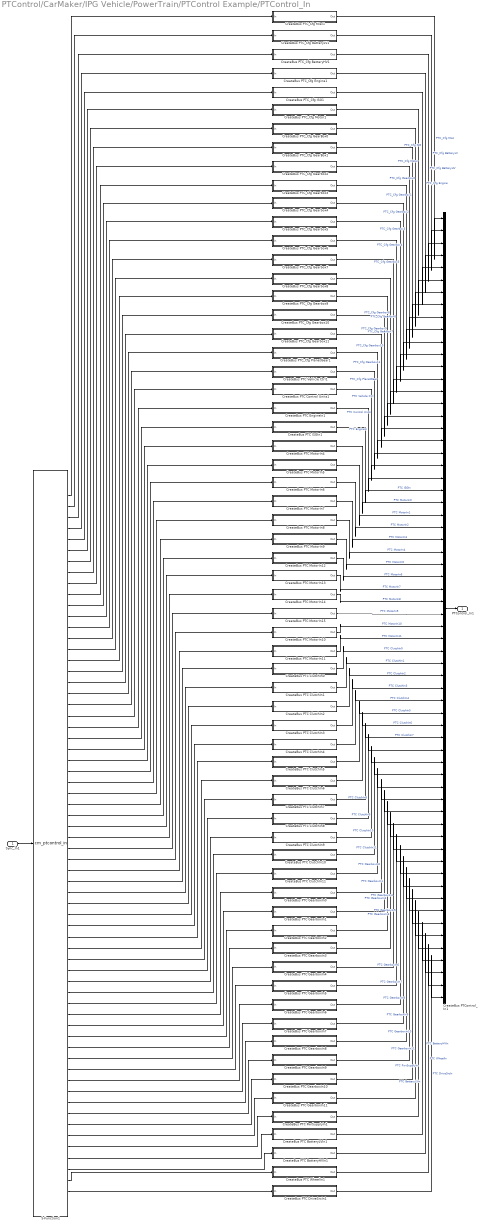
== system PTControl/CarMaker/IPG Vehicle/PowerTrain/PTControl Example/PTControl_In ==
  Sync_In1 : Inport
  CreateBus PTC BatteryHVIn1 : Subsystem
  CreateBus PTC BatteryLVIn1 : Subsystem
  CreateBus PTC ClutchIn0 : Subsystem
  CreateBus PTC ClutchIn1 : Subsystem
  CreateBus PTC ClutchIn10 : Subsystem
  CreateBus PTC ClutchIn11 : Subsystem
  CreateBus PTC ClutchIn2 : Subsystem
  CreateBus PTC ClutchIn3 : Subsystem
  CreateBus PTC ClutchIn4 : Subsystem
  CreateBus PTC ClutchIn5 : Subsystem
  CreateBus PTC ClutchIn6 : Subsystem
  CreateBus PTC ClutchIn7 : Subsystem
  CreateBus PTC ClutchIn8 : Subsystem
  CreateBus PTC ClutchIn9 : Subsystem
  CreateBus PTC Control Units1 : Subsystem
  CreateBus PTC DriveSrcIn1 : Subsystem
  CreateBus PTC EngineIn1 : Subsystem
  CreateBus PTC GearboxIn0 : Subsystem
  CreateBus PTC GearboxIn1 : Subsystem
  CreateBus PTC GearboxIn10 : Subsystem
  CreateBus PTC GearboxIn11 : Subsystem
  CreateBus PTC GearboxIn2 : Subsystem
  CreateBus PTC GearboxIn3 : Subsystem
  CreateBus PTC GearboxIn4 : Subsystem
  CreateBus PTC GearboxIn5 : Subsystem
  CreateBus PTC GearboxIn6 : Subsystem
  CreateBus PTC GearboxIn7 : Subsystem
  CreateBus PTC GearboxIn8 : Subsystem
  CreateBus PTC GearboxIn9 : Subsystem
  CreateBus PTC ISGIn1 : Subsystem
  CreateBus PTC MotorIn10 : Subsystem
  CreateBus PTC MotorIn11 : Subsystem
  CreateBus PTC MotorIn12 : Subsystem
  CreateBus PTC MotorIn13 : Subsystem
  CreateBus PTC MotorIn14 : Subsystem
  CreateBus PTC MotorIn15 : Subsystem
  CreateBus PTC MotorIn4 : Subsystem
  CreateBus PTC MotorIn5 : Subsystem
  CreateBus PTC MotorIn6 : Subsystem
  CreateBus PTC MotorIn7 : Subsystem
  CreateBus PTC MotorIn8 : Subsystem
  CreateBus PTC MotorIn9 : Subsystem
  CreateBus PTC PwrSupplyIn1 : Subsystem
  CreateBus PTC Vehicle Ctrl1 : Subsystem
  CreateBus PTC WheelIn1 : Subsystem
  CreateBus PTC_Cfg BatteryHV1 : Subsystem
  CreateBus PTC_Cfg BatteryLV1 : Subsystem
  CreateBus PTC_Cfg Engine1 : Subsystem
  CreateBus PTC_Cfg GearBox0 : Subsystem
  CreateBus PTC_Cfg GearBox1 : Subsystem
  CreateBus PTC_Cfg Gearbox10 : Subsystem
  CreateBus PTC_Cfg Gearbox11 : Subsystem
  CreateBus PTC_Cfg Gearbox2 : Subsystem
  CreateBus PTC_Cfg Gearbox3 : Subsystem
  CreateBus PTC_Cfg Gearbox4 : Subsystem
  CreateBus PTC_Cfg Gearbox5 : Subsystem
  CreateBus PTC_Cfg Gearbox6 : Subsystem
  CreateBus PTC_Cfg Gearbox7 : Subsystem
  CreateBus PTC_Cfg Gearbox8 : Subsystem
  CreateBus PTC_Cfg Gearbox9 : Subsystem
  CreateBus PTC_Cfg ISG1 : Subsystem
  CreateBus PTC_Cfg Misc1 : Subsystem
  CreateBus PTC_Cfg Motor1 : Subsystem
  CreateBus PTC_Cfg PlanetGear1 : Subsystem
  CreateBus PTControl_In1 : BusCreator  Inputs=64
  S-Function1 : S-Function  FunctionName=cm_ptcontrol_in  SFunctionDeploymentMode=off  EnableBusSupport=off
  PTControl_In1 : Outport  VectorParamsAs1DForOutWhenUnconnected=off
  wires:
  CreateBus PTC MotorIn8/1(Out) -> CreateBus PTControl_In1/28  "PTC MotorIn4"
  CreateBus PTC MotorIn15/1(Out) -> CreateBus PTControl_In1/33  "PTC MotorIn9"
  CreateBus PTC GearboxIn1/1(Out) -> CreateBus PTControl_In1/49  "PTC GearboxIn1"
  CreateBus PTC_Cfg BatteryHV1/1(Out) -> CreateBus PTControl_In1/3  "PTC_Cfg BatteryHV"
  CreateBus PTC ClutchIn7/1(Out) -> CreateBus PTControl_In1/43  "PTC ClutchIn7"
  S-Function1/56 -> CreateBus PTC GearboxIn8/1(In)
  CreateBus PTC_Cfg GearBox0/1(Out) -> CreateBus PTControl_In1/7  "PTC_Cfg Gearbox0"
  S-Function1/51 -> CreateBus PTC GearboxIn3/1(In)
  S-Function1/16 -> CreateBus PTC_Cfg Gearbox9/1(In)
  S-Function1/43 -> CreateBus PTC ClutchIn7/1(In)
  CreateBus PTC ClutchIn0/1(Out) -> CreateBus PTControl_In1/36  "PTC ClutchIn0"
  CreateBus PTC GearboxIn4/1(Out) -> CreateBus PTControl_In1/52  "PTC GearboxIn4"
  CreateBus PTC_Cfg Engine1/1(Out) -> CreateBus PTControl_In1/4  "PTC_Cfg Engine"
  CreateBus PTC GearboxIn7/1(Out) -> CreateBus PTControl_In1/55  "PTC GearboxIn7"
  CreateBus PTC_Cfg BatteryLV1/1(Out) -> CreateBus PTControl_In1/2  "PTC_Cfg BatteryLV"
  S-Function1/31 -> CreateBus PTC MotorIn13/1(In)
  CreateBus PTC_Cfg Gearbox7/1(Out) -> CreateBus PTControl_In1/14  "PTC_Cfg Gearbox7"
  CreateBus PTC GearboxIn5/1(Out) -> CreateBus PTControl_In1/53  "PTC GearboxIn5"
  CreateBus PTC_Cfg GearBox1/1(Out) -> CreateBus PTControl_In1/8  "PTC_Cfg Gearbox1"
  S-Function1/48 -> CreateBus PTC GearboxIn0/1(In)
  CreateBus PTC EngineIn1/1(Out) -> CreateBus PTControl_In1/22  "PTC EngineIn"
  S-Function1/39 -> CreateBus PTC ClutchIn3/1(In)
  S-Function1/4 -> CreateBus PTC_Cfg Engine1/1(In)
  CreateBus PTC BatteryLVIn1/1(Out) -> CreateBus PTControl_In1/61  "PTC BatteryLVIn"
  CreateBus PTControl_In1/1 -> PTControl_In1/1
  S-Function1/15 -> CreateBus PTC_Cfg Gearbox8/1(In)
  CreateBus PTC_Cfg Motor1/1(Out) -> CreateBus PTControl_In1/6  "PTC_Cfg Motor"
  CreateBus PTC MotorIn13/1(Out) -> CreateBus PTControl_In1/31  "PTC MotorIn7"
  S-Function1/46 -> CreateBus PTC ClutchIn10/1(In)
  CreateBus PTC DriveSrcIn1/1(Out) -> CreateBus PTControl_In1/64  "PTC DriveSrcIn"
  S-Function1/21 -> CreateBus PTC Control Units1/1(In)
  S-Function1/30 -> CreateBus PTC MotorIn12/1(In)
  S-Function1/19 -> CreateBus PTC_Cfg PlanetGear1/1(In)
  CreateBus PTC MotorIn5/1(Out) -> CreateBus PTControl_In1/25  "PTC MotorIn1"
  S-Function1/40 -> CreateBus PTC ClutchIn4/1(In)
  S-Function1/3 -> CreateBus PTC_Cfg BatteryHV1/1(In)
  CreateBus PTC MotorIn6/1(Out) -> CreateBus PTControl_In1/26  "PTC MotorIn2"
  S-Function1/47 -> CreateBus PTC ClutchIn11/1(In)
  CreateBus PTC MotorIn7/1(Out) -> CreateBus PTControl_In1/27  "PTC MotorIn3"
  S-Function1/18 -> CreateBus PTC_Cfg Gearbox11/1(In)
  CreateBus PTC ClutchIn3/1(Out) -> CreateBus PTControl_In1/39  "PTC ClutchIn3"
  S-Function1/55 -> CreateBus PTC GearboxIn7/1(In)
  S-Function1/63 -> CreateBus PTC WheelIn1/1(In)
  S-Function1/25 -> CreateBus PTC MotorIn5/1(In)
  Sync_In1/1 -> S-Function1/1
  S-Function1/14 -> CreateBus PTC_Cfg Gearbox7/1(In)
  CreateBus PTC ClutchIn1/1(Out) -> CreateBus PTControl_In1/37  "PTC ClutchIn1"
  S-Function1/1 -> CreateBus PTC_Cfg Misc1/1(In)
  CreateBus PTC GearboxIn10/1(Out) -> CreateBus PTControl_In1/58  "PTC GearboxIn10"
  S-Function1/49 -> CreateBus PTC GearboxIn1/1(In)
  S-Function1/37 -> CreateBus PTC ClutchIn1/1(In)
  CreateBus PTC ClutchIn10/1(Out) -> CreateBus PTControl_In1/46  "PTC ClutchIn10"
  S-Function1/28 -> CreateBus PTC MotorIn8/1(In)
  CreateBus PTC GearboxIn0/1(Out) -> CreateBus PTControl_In1/48  "PTC GearboxIn0"
  CreateBus PTC GearboxIn9/1(Out) -> CreateBus PTControl_In1/57  "PTC GearboxIn9"
  S-Function1/36 -> CreateBus PTC ClutchIn0/1(In)
  S-Function1/12 -> CreateBus PTC_Cfg Gearbox5/1(In)
  CreateBus PTC_Cfg PlanetGear1/1(Out) -> CreateBus PTControl_In1/19  "PTC_Cfg PlanetGear"
  CreateBus PTC ClutchIn6/1(Out) -> CreateBus PTControl_In1/42  "PTC ClutchIn6"
  CreateBus PTC MotorIn12/1(Out) -> CreateBus PTControl_In1/30  "PTC MotorIn6"
  S-Function1/38 -> CreateBus PTC ClutchIn2/1(In)
  CreateBus PTC_Cfg Gearbox6/1(Out) -> CreateBus PTControl_In1/13  "PTC_Cfg Gearbox6"
  S-Function1/44 -> CreateBus PTC ClutchIn8/1(In)
  CreateBus PTC_Cfg Gearbox2/1(Out) -> CreateBus PTControl_In1/9  "PTC_Cfg Gearbox2"
  CreateBus PTC Vehicle Ctrl1/1(Out) -> CreateBus PTControl_In1/20  "PTC Vehicle Ctrl"
  CreateBus PTC GearboxIn11/1(Out) -> CreateBus PTControl_In1/59  "PTC GearboxIn11"
  S-Function1/29 -> CreateBus PTC MotorIn9/1(In)
  S-Function1/34 -> CreateBus PTC MotorIn10/1(In)
  S-Function1/58 -> CreateBus PTC GearboxIn10/1(In)
  S-Function1/8 -> CreateBus PTC_Cfg GearBox1/1(In)
  S-Function1/57 -> CreateBus PTC GearboxIn9/1(In)
  CreateBus PTC GearboxIn8/1(Out) -> CreateBus PTControl_In1/56  "PTC GearboxIn8"
  S-Function1/62 -> CreateBus PTC BatteryHVIn1/1(In)
  CreateBus PTC GearboxIn2/1(Out) -> CreateBus PTControl_In1/50  "PTC GearboxIn2"
  CreateBus PTC MotorIn11/1(Out) -> CreateBus PTControl_In1/35  "PTC MotorIn11"
  S-Function1/32 -> CreateBus PTC MotorIn14/1(In)
  S-Function1/27 -> CreateBus PTC MotorIn7/1(In)
  S-Function1/11 -> CreateBus PTC_Cfg Gearbox4/1(In)
  CreateBus PTC MotorIn10/1(Out) -> CreateBus PTControl_In1/34  "PTC MotorIn10"
  CreateBus PTC ClutchIn11/1(Out) -> CreateBus PTControl_In1/47  "PTC ClutchIn11"
  S-Function1/64 -> CreateBus PTC DriveSrcIn1/1(In)
  CreateBus PTC MotorIn14/1(Out) -> CreateBus PTControl_In1/32  "PTC MotorIn8"
  CreateBus PTC ClutchIn9/1(Out) -> CreateBus PTControl_In1/45  "PTC ClutchIn9"
  S-Function1/59 -> CreateBus PTC GearboxIn11/1(In)
  CreateBus PTC_Cfg Gearbox4/1(Out) -> CreateBus PTControl_In1/11  "PTC_Cfg Gearbox4"
  S-Function1/61 -> CreateBus PTC BatteryLVIn1/1(In)
  S-Function1/41 -> CreateBus PTC ClutchIn5/1(In)
  S-Function1/23 -> CreateBus PTC ISGIn1/1(In)
  S-Function1/13 -> CreateBus PTC_Cfg Gearbox6/1(In)
  S-Function1/7 -> CreateBus PTC_Cfg GearBox0/1(In)
  S-Function1/50 -> CreateBus PTC GearboxIn2/1(In)
  S-Function1/52 -> CreateBus PTC GearboxIn4/1(In)
  CreateBus PTC ClutchIn2/1(Out) -> CreateBus PTControl_In1/38  "PTC ClutchIn2"
  CreateBus PTC_Cfg Misc1/1(Out) -> CreateBus PTControl_In1/1  "PTC_Cfg Misc"
  S-Function1/17 -> CreateBus PTC_Cfg Gearbox10/1(In)
  S-Function1/33 -> CreateBus PTC MotorIn15/1(In)
  CreateBus PTC_Cfg ISG1/1(Out) -> CreateBus PTControl_In1/5  "PTC_Cfg ISG"
  S-Function1/20 -> CreateBus PTC Vehicle Ctrl1/1(In)
  S-Function1/35 -> CreateBus PTC MotorIn11/1(In)
  CreateBus PTC PwrSupplyIn1/1(Out) -> CreateBus PTControl_In1/60  "PTC PwrSupplyIn"
  CreateBus PTC MotorIn9/1(Out) -> CreateBus PTControl_In1/29  "PTC MotorIn5"
  CreateBus PTC ClutchIn8/1(Out) -> CreateBus PTControl_In1/44  "PTC ClutchIn8"
  S-Function1/53 -> CreateBus PTC GearboxIn5/1(In)
  S-Function1/6 -> CreateBus PTC_Cfg Motor1/1(In)
  CreateBus PTC_Cfg Gearbox5/1(Out) -> CreateBus PTControl_In1/12  "PTC_Cfg Gearbox5"
  CreateBus PTC Control Units1/1(Out) -> CreateBus PTControl_In1/21  "PTC Control Units"
  S-Function1/26 -> CreateBus PTC MotorIn6/1(In)
  CreateBus PTC GearboxIn3/1(Out) -> CreateBus PTControl_In1/51  "PTC GearboxIn3"
  CreateBus PTC ClutchIn5/1(Out) -> CreateBus PTControl_In1/41  "PTC ClutchIn5"
  S-Function1/24 -> CreateBus PTC MotorIn4/1(In)
  CreateBus PTC_Cfg Gearbox8/1(Out) -> CreateBus PTControl_In1/15  "PTC_Cfg Gearbox8"
  S-Function1/10 -> CreateBus PTC_Cfg Gearbox3/1(In)
  S-Function1/5 -> CreateBus PTC_Cfg ISG1/1(In)
  CreateBus PTC WheelIn1/1(Out) -> CreateBus PTControl_In1/63  "PTC WheelIn"
  CreateBus PTC ISGIn1/1(Out) -> CreateBus PTControl_In1/23  "PTC ISGIn"
  CreateBus PTC_Cfg Gearbox10/1(Out) -> CreateBus PTControl_In1/17  "PTC_Cfg Gearbox10"
  CreateBus PTC ClutchIn4/1(Out) -> CreateBus PTControl_In1/40  "PTC ClutchIn4"
  S-Function1/2 -> CreateBus PTC_Cfg BatteryLV1/1(In)
  CreateBus PTC_Cfg Gearbox3/1(Out) -> CreateBus PTControl_In1/10  "PTC_Cfg Gearbox3"
  S-Function1/42 -> CreateBus PTC ClutchIn6/1(In)
  S-Function1/54 -> CreateBus PTC GearboxIn6/1(In)
  CreateBus PTC GearboxIn6/1(Out) -> CreateBus PTControl_In1/54  "PTC GearboxIn6"
  S-Function1/9 -> CreateBus PTC_Cfg Gearbox2/1(In)
  CreateBus PTC MotorIn4/1(Out) -> CreateBus PTControl_In1/24  "PTC MotorIn0"
  S-Function1/60 -> CreateBus PTC PwrSupplyIn1/1(In)
  CreateBus PTC BatteryHVIn1/1(Out) -> CreateBus PTControl_In1/62  "PTC BatteryHVIn"
  CreateBus PTC_Cfg Gearbox11/1(Out) -> CreateBus PTControl_In1/18  "PTC_Cfg Gearbox11"
  CreateBus PTC_Cfg Gearbox9/1(Out) -> CreateBus PTControl_In1/16  "PTC_Cfg Gearbox9"
  S-Function1/45 -> CreateBus PTC ClutchIn9/1(In)
  S-Function1/22 -> CreateBus PTC EngineIn1/1(In)

== system PTControl/CarMaker/IPG Vehicle/PowerTrain/PTControl Example/PTControl_Out1 ==
  PTC MiscOut : Inport
  PTC EngineOut : Inport  Port=2
  PTC ISGOut : Inport  Port=3
  PTC MotorOut : Inport  Port=4
  PTC ClutchOut : Inport  Port=5
  PTC GearboxOut : Inport  Port=6
  PTC PwrSupplyOut : Inport  Port=7
  PTC BattLV_Out : Inport  Port=8
  PTC BattHV_Out : Inport  Port=9
  PTC WheelOut : Inport  Port=10
  Bus Selector1 : BusSelector  OutputSignals=PTC MotorOut0,PTC MotorOut1,PTC MotorOut2,PTC MotorOut3,PTC MotorOut4,PTC MotorOut5,PTC MotorOut6,PTC MotorOut7,PTC MotorOut8,PTC MotorOut9,PTC MotorOut10,PTC MotorOut11
  Bus Selector2 : BusSelector  OutputSignals=PTC ClutchOut0,PTC ClutchOut1,PTC ClutchOut2,PTC ClutchOut3,PTC ClutchOut4,PTC ClutchOut5,PTC ClutchOut6,PTC ClutchOut7,PTC ClutchOut8,PTC ClutchOut9,PTC ClutchOut10,PTC ClutchOut11
  Bus Selector3 : BusSelector  OutputSignals=PTC GearBoxOut0,PTC GearBoxOut1,PTC GearBoxOut2,PTC GearBoxOut3,PTC GearBoxOut4,PTC GearBoxOut5,PTC GearBoxOut6,PTC GearBoxOut7,PTC GearBoxOut8,PTC GearBoxOut9,PTC GearBoxOut10,PTC GearBoxOut11
  PTControl_Out : S-Function  FunctionName=cm_ptcontrol_out  SFunctionDeploymentMode=off  EnableBusSupport=off
  wires:
  PTC MotorOut/1 -> Bus Selector1/1
  PTC ISGOut/1 -> PTControl_Out/3
  PTC EngineOut/1 -> PTControl_Out/2
  PTC MiscOut/1 -> PTControl_Out/1
  Bus Selector1/1 -> PTControl_Out/4  "<PTC MotorOut0>"
  Bus Selector1/2 -> PTControl_Out/5  "<PTC MotorOut1>"
  Bus Selector1/3 -> PTControl_Out/6  "<PTC MotorOut2>"
  Bus Selector1/4 -> PTControl_Out/7  "<PTC MotorOut3>"
  Bus Selector1/5 -> PTControl_Out/8  "<PTC MotorOut4>"
  Bus Selector1/6 -> PTControl_Out/9  "<PTC MotorOut5>"
  Bus Selector1/7 -> PTControl_Out/10  "<PTC MotorOut6>"
  Bus Selector1/8 -> PTControl_Out/11  "<PTC MotorOut7>"
  Bus Selector1/9 -> PTControl_Out/12  "<PTC MotorOut8>"
  Bus Selector1/10 -> PTControl_Out/13  "<PTC MotorOut9>"
  Bus Selector1/11 -> PTControl_Out/14  "<PTC MotorOut10>"
  Bus Selector1/12 -> PTControl_Out/15  "<PTC MotorOut11>"
  PTC ClutchOut/1 -> Bus Selector2/1
  Bus Selector2/1 -> PTControl_Out/16  "<PTC ClutchOut0>"
  Bus Selector2/2 -> PTControl_Out/17  "<PTC ClutchOut1>"
  Bus Selector2/3 -> PTControl_Out/18  "<PTC ClutchOut2>"
  Bus Selector2/4 -> PTControl_Out/19  "<PTC ClutchOut3>"
  Bus Selector2/5 -> PTControl_Out/20  "<PTC ClutchOut4>"
  Bus Selector2/6 -> PTControl_Out/21  "<PTC ClutchOut5>"
  Bus Selector2/7 -> PTControl_Out/22  "<PTC ClutchOut6>"
  Bus Selector2/8 -> PTControl_Out/23  "<PTC ClutchOut7>"
  Bus Selector2/9 -> PTControl_Out/24  "<PTC ClutchOut8>"
  Bus Selector2/10 -> PTControl_Out/25  "<PTC ClutchOut9>"
  Bus Selector2/11 -> PTControl_Out/26  "<PTC ClutchOut10>"
  Bus Selector2/12 -> PTControl_Out/27  "<PTC ClutchOut11>"
  PTC GearboxOut/1 -> Bus Selector3/1
  Bus Selector3/1 -> PTControl_Out/28  "<PTC GearBoxOut0>"
  Bus Selector3/2 -> PTControl_Out/29  "<PTC GearBoxOut1>"
  Bus Selector3/3 -> PTControl_Out/30  "<PTC GearBoxOut2>"
  Bus Selector3/4 -> PTControl_Out/31  "<PTC GearBoxOut3>"
  Bus Selector3/5 -> PTControl_Out/32  "<PTC GearBoxOut4>"
  Bus Selector3/6 -> PTControl_Out/33  "<PTC GearBoxOut5>"
  Bus Selector3/7 -> PTControl_Out/34  "<PTC GearBoxOut6>"
  Bus Selector3/8 -> PTControl_Out/35  "<PTC GearBoxOut7>"
  Bus Selector3/9 -> PTControl_Out/36  "<PTC GearBoxOut8>"
  Bus Selector3/10 -> PTControl_Out/37  "<PTC GearBoxOut9>"
  Bus Selector3/11 -> PTControl_Out/38  "<PTC GearBoxOut10>"
  Bus Selector3/12 -> PTControl_Out/39  "<PTC GearBoxOut11>"
  PTC PwrSupplyOut/1 -> PTControl_Out/40
  PTC BattLV_Out/1 -> PTControl_Out/41
  PTC BattHV_Out/1 -> PTControl_Out/42
  PTC WheelOut/1 -> PTControl_Out/43

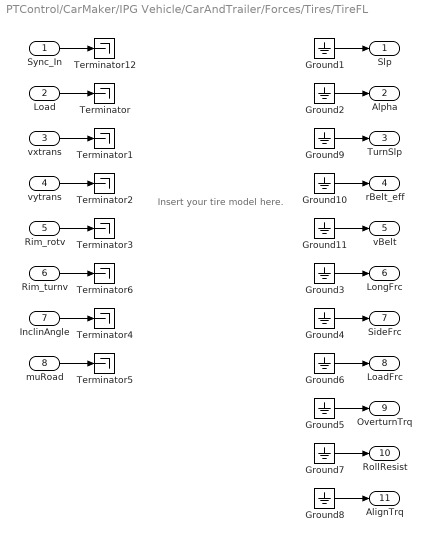
== system PTControl/CarMaker/IPG Vehicle/CarAndTrailer/Forces/Tires/TireFL ==
  note: Insert your tire model here.
  Sync_In : Inport
  Load : Inport  Port=2
  vxtrans : Inport  Port=3
  vytrans : Inport  Port=4
  Rim_rotv : Inport  Port=5
  Rim_turnv : Inport  Port=6
  InclinAngle : Inport  Port=7
  muRoad : Inport  Port=8
  Ground{1..11} (11 alike) : Ground
  Terminator{,1..6,12} (8 alike) : Terminator
  Slp : Outport  VectorParamsAs1DForOutWhenUnconnected=off
  Alpha : Outport  Port=2  VectorParamsAs1DForOutWhenUnconnected=off
  TurnSlp : Outport  Port=3  VectorParamsAs1DForOutWhenUnconnected=off
  rBelt_eff : Outport  Port=4  VectorParamsAs1DForOutWhenUnconnected=off
  vBelt : Outport  Port=5  VectorParamsAs1DForOutWhenUnconnected=off
  LongFrc : Outport  Port=6  VectorParamsAs1DForOutWhenUnconnected=off
  SideFrc : Outport  Port=7  VectorParamsAs1DForOutWhenUnconnected=off
  LoadFrc : Outport  Port=8  VectorParamsAs1DForOutWhenUnconnected=off
  OverturnTrq : Outport  Port=9  VectorParamsAs1DForOutWhenUnconnected=off
  RollResist : Outport  Port=10  VectorParamsAs1DForOutWhenUnconnected=off
  AlignTrq : Outport  Port=11  VectorParamsAs1DForOutWhenUnconnected=off
  wires:
  Ground11/1 -> vBelt/1
  Ground10/1 -> rBelt_eff/1
  Ground9/1 -> TurnSlp/1
  Rim_turnv/1 -> Terminator6/1
  Sync_In/1 -> Terminator12/1
  Ground2/1 -> Alpha/1
  Ground3/1 -> LongFrc/1
  Ground4/1 -> SideFrc/1
  Ground5/1 -> OverturnTrq/1
  vxtrans/1 -> Terminator1/1
  vytrans/1 -> Terminator2/1
  Rim_rotv/1 -> Terminator3/1
  InclinAngle/1 -> Terminator4/1
  muRoad/1 -> Terminator5/1
  Load/1 -> Terminator/1
  Ground1/1 -> Slp/1
  Ground6/1 -> LoadFrc/1
  Ground7/1 -> RollResist/1
  Ground8/1 -> AlignTrq/1

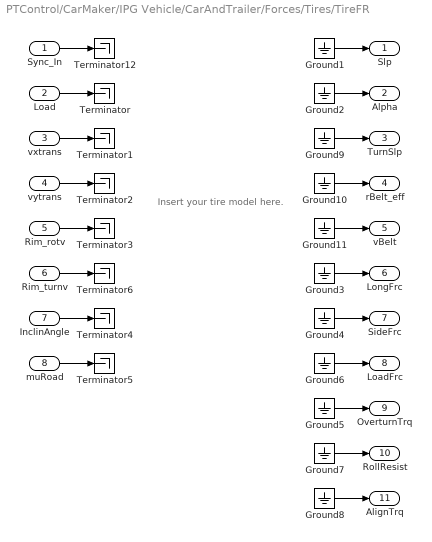
== system PTControl/CarMaker/IPG Vehicle/CarAndTrailer/Forces/Tires/TireFR ==
  note: Insert your tire model here.
  Sync_In : Inport
  Load : Inport  Port=2
  vxtrans : Inport  Port=3
  vytrans : Inport  Port=4
  Rim_rotv : Inport  Port=5
  Rim_turnv : Inport  Port=6
  InclinAngle : Inport  Port=7
  muRoad : Inport  Port=8
  Ground{1..11} (11 alike) : Ground
  Terminator{,1..6,12} (8 alike) : Terminator
  Slp : Outport  VectorParamsAs1DForOutWhenUnconnected=off
  Alpha : Outport  Port=2  VectorParamsAs1DForOutWhenUnconnected=off
  TurnSlp : Outport  Port=3  VectorParamsAs1DForOutWhenUnconnected=off
  rBelt_eff : Outport  Port=4  VectorParamsAs1DForOutWhenUnconnected=off
  vBelt : Outport  Port=5  VectorParamsAs1DForOutWhenUnconnected=off
  LongFrc : Outport  Port=6  VectorParamsAs1DForOutWhenUnconnected=off
  SideFrc : Outport  Port=7  VectorParamsAs1DForOutWhenUnconnected=off
  LoadFrc : Outport  Port=8  VectorParamsAs1DForOutWhenUnconnected=off
  OverturnTrq : Outport  Port=9  VectorParamsAs1DForOutWhenUnconnected=off
  RollResist : Outport  Port=10  VectorParamsAs1DForOutWhenUnconnected=off
  AlignTrq : Outport  Port=11  VectorParamsAs1DForOutWhenUnconnected=off
  wires:
  Ground11/1 -> vBelt/1
  Ground10/1 -> rBelt_eff/1
  Ground9/1 -> TurnSlp/1
  Rim_turnv/1 -> Terminator6/1
  Sync_In/1 -> Terminator12/1
  Ground2/1 -> Alpha/1
  Ground3/1 -> LongFrc/1
  Ground4/1 -> SideFrc/1
  Ground5/1 -> OverturnTrq/1
  vxtrans/1 -> Terminator1/1
  vytrans/1 -> Terminator2/1
  Rim_rotv/1 -> Terminator3/1
  InclinAngle/1 -> Terminator4/1
  muRoad/1 -> Terminator5/1
  Load/1 -> Terminator/1
  Ground1/1 -> Slp/1
  Ground6/1 -> LoadFrc/1
  Ground7/1 -> RollResist/1
  Ground8/1 -> AlignTrq/1

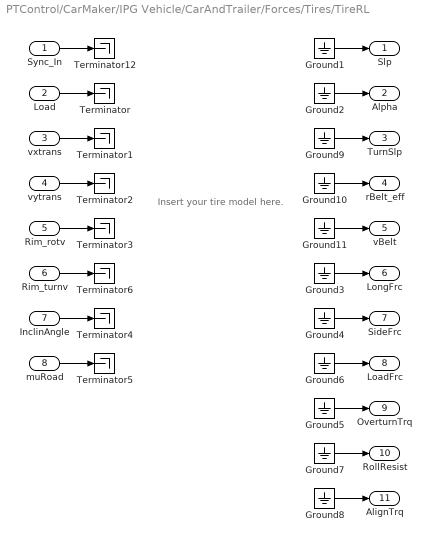
== system PTControl/CarMaker/IPG Vehicle/CarAndTrailer/Forces/Tires/TireRL ==
  note: Insert your tire model here.
  Sync_In : Inport
  Load : Inport  Port=2
  vxtrans : Inport  Port=3
  vytrans : Inport  Port=4
  Rim_rotv : Inport  Port=5
  Rim_turnv : Inport  Port=6
  InclinAngle : Inport  Port=7
  muRoad : Inport  Port=8
  Ground{1..11} (11 alike) : Ground
  Terminator{,1..6,12} (8 alike) : Terminator
  Slp : Outport  VectorParamsAs1DForOutWhenUnconnected=off
  Alpha : Outport  Port=2  VectorParamsAs1DForOutWhenUnconnected=off
  TurnSlp : Outport  Port=3  VectorParamsAs1DForOutWhenUnconnected=off
  rBelt_eff : Outport  Port=4  VectorParamsAs1DForOutWhenUnconnected=off
  vBelt : Outport  Port=5  VectorParamsAs1DForOutWhenUnconnected=off
  LongFrc : Outport  Port=6  VectorParamsAs1DForOutWhenUnconnected=off
  SideFrc : Outport  Port=7  VectorParamsAs1DForOutWhenUnconnected=off
  LoadFrc : Outport  Port=8  VectorParamsAs1DForOutWhenUnconnected=off
  OverturnTrq : Outport  Port=9  VectorParamsAs1DForOutWhenUnconnected=off
  RollResist : Outport  Port=10  VectorParamsAs1DForOutWhenUnconnected=off
  AlignTrq : Outport  Port=11  VectorParamsAs1DForOutWhenUnconnected=off
  wires:
  Ground11/1 -> vBelt/1
  Ground10/1 -> rBelt_eff/1
  Ground9/1 -> TurnSlp/1
  Rim_turnv/1 -> Terminator6/1
  Sync_In/1 -> Terminator12/1
  Ground2/1 -> Alpha/1
  Ground3/1 -> LongFrc/1
  Ground4/1 -> SideFrc/1
  Ground5/1 -> OverturnTrq/1
  vxtrans/1 -> Terminator1/1
  vytrans/1 -> Terminator2/1
  Rim_rotv/1 -> Terminator3/1
  InclinAngle/1 -> Terminator4/1
  muRoad/1 -> Terminator5/1
  Load/1 -> Terminator/1
  Ground1/1 -> Slp/1
  Ground6/1 -> LoadFrc/1
  Ground7/1 -> RollResist/1
  Ground8/1 -> AlignTrq/1
